simulink model "for_elsa"  (R2020a)
settings: Solver=FixedStepAuto  StartTime=0.0  StopTime=10.0  FixedStep=1e-3  RelTol=1e-3  EnableMultiTasking=on
undefined symbols (not defined in the file): A0, A1, D0, D1, D10, D11, D12, D13, D2, D3, D4, D5, D6, D7, D8, D9, PTA0, PTA1, PTA2, PTB2, PTB23, PTB3, PTB9, PTC16, PTC17, PTC2, PTC3, PTC4, PTD0, PTD1, PTD2, PTD3
libraries: frdmk64flib x22, etargetslib x16, dspstat3 x1
settings Model: ExtModeTrigDuration=5  Creator=Luis  LastModifiedBy=Steven
settings OptimizationCC: EnhancedBackFolding=on  PassReuseOutputArgsAs=Individual arguments  ZeroExternalMemoryAtStartup=off  ZeroInternalMemoryAtStartup=off  MaxStackSize=64  OptimizeBlockOrder=speed  DifferentSizesBufferReuse=on  OptimizationCustomize=off  EfficientTunableParamExpr=on
settings DebuggingCC: ParameterTunabilityLossMsg=error
settings HardwareCC: ProdBitPerPointer=32  ProdBitPerSizeT=32  ProdBitPerPtrDiffT=32  ProdLargestAtomicInteger=Long  ProdLargestAtomicFloat=Double  ProdWordSize=32  ProdHWDeviceType=ARM Compatible->ARM Cortex
settings SFSimCC: MATLABDynamicMemAlloc=off
settings RTWCC: SystemTargetFile=ert.tlc  HardwareBoard=NXP FRDM-K64F  TemplateMakefile=ert_default_tmf  Toolchain=GNU Tools for ARM Embedded Processors
settings CodeAppCC: ForceParamTrailComments=on  IgnoreCustomStorageClasses=off  OperatorAnnotations=on  SimulinkDataObjDesc=on  SFDataObjDesc=on  InsertBlockDesc=on

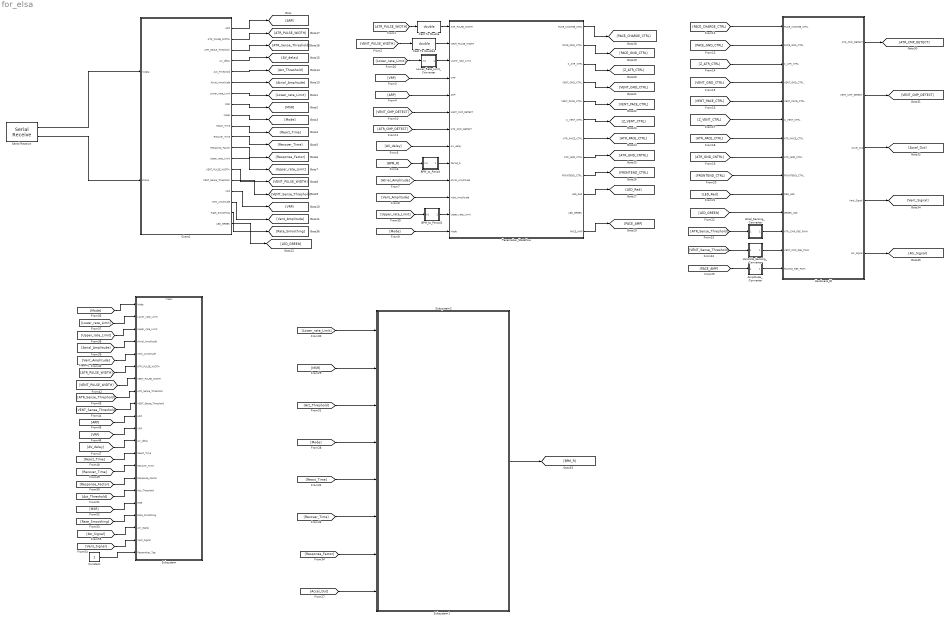
== system for_elsa ==
  Amplitude_Converter : Subsystem
  Atrial_Sensing_Converter : Subsystem
  BPM_to_Period : Subsystem
  BPM_to_Period1 : Subsystem
  Cast To Double : DataTypeConversion  OutDataTypeStr=double
  Cast To Double1 : DataTypeConversion  OutDataTypeStr=double
  Chart1 : Stateflow chart  TreatAsAtomicUnit=on
  Constant : Constant  OutDataTypeStr=uint8
  Hardware_IO : Subsystem
  Lower_Rate_Limit_Converter : Subsystem
  "Pacemaker_Stateflow " : Stateflow chart  TreatAsAtomicUnit=on
      settings: PortSchema="{\"entries\":[{\"content\":{\"sides\":[{\"content\":{\"connectorIds\":[\"In1\",\"In4\",\"In2\",\"In5\",\"In6\",\"In7\",\"In8\",\"In9\",\"In10\",\"In11\",\"In12\",\"In13\",\"In3\"]},\"type\":\"ConnectorPlacement.EquallySpacedRectSide\",\"uuid\":\"f97b12ff-cb00-4386-a373-7143c3a8b48d\"},{\"content\":{\"connectorIds\":[\"Out1\",\"Out2\",\"Out3\",\"Out4\",\"Out5\",\"Out6\",\"Out7\",\"Out8\",\"Out9\",\"Out10\",\"Out11\",\"Out12\"],\"side\":\"RIGHT\"},\"type\":\"ConnectorPlacement.EquallySpacedRectSide\",\"uuid\":\"90163773-f9d1-46de-bd72-9589b8539202\"},{\"content\":{\"connectorIds\":[],\"side\":\"TOP\"},\"type\":\"ConnectorPlacement.EquallySpacedRectSide\",\"uuid\":\"f8a54119-a7c4-4071-8260-df405210e670\"},{\"content\":{\"connectorIds\":[],\"side\":\"BOTTOM\"},\"type\":\"ConnectorPlacement.EquallySpacedRectSide\",\"uuid\":\"70f9d800-d0b8-46e1-812e-9f4712f7acbd\"}]},\"type\":\"ConnectorPlacement.EquallySpacedConnector\",\"uuid\":\"47f7c40c-c42b-42f7-beed-99d299c6cdee\"}],\"packageUris\":[\"http://schema.mathworks.com/mf0/Connector/19700101\"],\"version\":\"1.0\"}"
  Serial Receive : frdmk64flib/Serial Receive  SCIModule=0  Baudrate=uint32(9600)  Parity=None  StopBits=1  HardwareFlowControl=None  ByteOrder=LittleEndian  DataType=uint8  DataLength=37  BlockingMode=off  OutputStatus=on  SampleTime=-1
  Subsystem : Subsystem
  Subsystem1 : Subsystem
  Subsystem2 : Subsystem
  Ventricle_Sensing_Converter : Subsystem
  wires:
  Lower_Rate_Limit_Converter/1(Out1) -> "Pacemaker_Stateflow "/2(Lower_rate_Limit)
  Ventricle_Sensing_Converter/1(Out1) -> Hardware_IO/13(VENT_CMP_REF_PWM)
  Amplitude_Converter/1(Out1) -> Hardware_IO/14(PACING_REF_PWM)
  Atrial_Sensing_Converter/1(Out1) -> Hardware_IO/12(ATR_CMP_REF_PWM)
  Chart1/1(ARP) -> [ARP]
  Chart1/17(Vent_Amplitude) -> [Vent_Amplitude]
  Chart1/16(VRP) -> [VRP]
  Chart1/15(VENT_Sense_Threshold) -> [VENT_Sense_Threshold]
  Chart1/14(VENT_PULSE_WIDTH) -> [VENT_PULSE_WIDTH]
  Chart1/13(Upper_rate_Limit) -> [Upper_rate_Limit]
  Chart1/12(Response_Factor) -> [Response_Factor]
  Chart1/11(Recover_Time) -> [Recover_Time]
  Chart1/10(React_Time) -> [React_Time]
  Chart1/9(Mode) -> [Mode]
  Chart1/8(MSR) -> [MSR]
  Chart1/7(Lower_rate_Limit) -> [Lower_rate_Limit]
  Chart1/5(Act_Threshold) -> [Act_Threshold]
  Chart1/6(Atrial_Amplitude) -> [Atrial_Amplitude]
  Chart1/4(AV_delay) -> [AV_delay]
  Chart1/3(ATR_Sense_Threshold) -> [ATR_Sense_Threshold]
  Chart1/2(ATR_PULSE_WIDTH) -> [ATR_PULSE_WIDTH]
  [Mode] -> "Pacemaker_Stateflow "/3(Mode)
  [Vent_Amplitude] -> "Pacemaker_Stateflow "/12(Vent_Amplitude)
  [Atrial_Amplitude] -> "Pacemaker_Stateflow "/11(Atrial_Amplitude)
  [BPM_R] -> BPM_to_Period/1(In1)
  [AV_delay] -> "Pacemaker_Stateflow "/9(AV_delay)
  [ARP] -> "Pacemaker_Stateflow "/6(ARP)
  [VRP] -> "Pacemaker_Stateflow "/5(VRP)
  [VENT_PULSE_WIDTH] -> Cast To Double1/1
  [ATR_PULSE_WIDTH] -> Cast To Double/1
  [ATR_CMP_DETECT] -> "Pacemaker_Stateflow "/8(ATR_CMP_DETECT)
  [VENT_CMP_DETECT] -> "Pacemaker_Stateflow "/7(VENT_CMP_DETECT)
  "Pacemaker_Stateflow "/1(PACE_CHARGE_CTRL) -> [PACE_CHARGE_CTRL]
  "Pacemaker_Stateflow "/2(PACE_GND_CTRL) -> [PACE_GND_CTRL]
  "Pacemaker_Stateflow "/3(Z_ATR_CTRL) -> [Z_ATR_CTRL]
  "Pacemaker_Stateflow "/4(VENT_GND_CTRL) -> [VENT_GND_CTRL]
  "Pacemaker_Stateflow "/5(VENT_PACE_CTRL) -> [VENT_PACE_CTRL]
  "Pacemaker_Stateflow "/6(Z_VENT_CTRL) -> [Z_VENT_CTRL]
  "Pacemaker_Stateflow "/7(ATR_PACE_CTRL) -> [ATR_PACE_CTRL]
  "Pacemaker_Stateflow "/8(ATR_GND_CTRL) -> [ATR_GND_CNTRL]
  "Pacemaker_Stateflow "/9(FRONTEND_CTRL) -> [FRONTEND_CTRL]
  "Pacemaker_Stateflow "/10(LED_Red) -> [LED_Red]
  "Pacemaker_Stateflow "/12(PACE_AMP) -> [PACE_AMP]
  [PACE_CHARGE_CTRL] -> Hardware_IO/1(PACE_CHARGE_CTRL)
  [PACE_GND_CTRL] -> Hardware_IO/2(PACE_GND_CTRL)
  [Z_ATR_CTRL] -> Hardware_IO/3(Z_ATR_CTRL)
  [VENT_GND_CTRL] -> Hardware_IO/4(VENT_GND_CTRL)
  [VENT_PACE_CTRL] -> Hardware_IO/5(VENT_PACE_CTRL)
  [Z_VENT_CTRL] -> Hardware_IO/6(Z_VENT_CTRL)
  [ATR_PACE_CTRL] -> Hardware_IO/7(ATR_PACE_CTRL)
  [ATR_GND_CNTRL] -> Hardware_IO/8(ATR_GND_CTRL)
  [FRONTEND_CTRL] -> Hardware_IO/9(FRONTEND_CTRL)
  [LED_Red] -> Hardware_IO/10(RED_LED)
  [LED_GREEN] -> Hardware_IO/11(GREEN_LED)
  Hardware_IO/1(ATR_CMP_DETECT) -> [ATR_CMP_DETECT]
  Hardware_IO/2(VENT_CMP_DETECT) -> [VENT_CMP_DETECT]
  [ATR_Sense_Threshold] -> Atrial_Sensing_Converter/1(In1)
  [VENT_Sense_Threshold] -> Ventricle_Sensing_Converter/1(In1)
  [PACE_AMP] -> Amplitude_Converter/1(In1)
  [Lower_rate_Limit] -> Lower_Rate_Limit_Converter/1(In1)
  BPM_to_Period/1(Out1) -> "Pacemaker_Stateflow "/10(Period_R)
  Hardware_IO/3(Accel_Out) -> [Accel_Out]
  [Lower_rate_Limit] -> Subsystem1/1(Lower_Rate)
  [MSR] -> Subsystem1/2(MSR)
  [Act_Threshold] -> Subsystem1/3(Activity_Thresh)
  [React_Time] -> Subsystem1/5(Reaction)
  [Recover_Time] -> Subsystem1/6(Recovery)
  [Response_Factor] -> Subsystem1/7(Response_Factor)
  [Accel_Out] -> Subsystem1/8(Accel_Out)
  Subsystem1/1(BPM_R) -> [BPM_R]
  [Mode] -> Subsystem1/4(Mode)
  Hardware_IO/4(Vent_Signal) -> [Vent_Signal]
  Hardware_IO/5(Atr_Signal) -> [Atr_Signal]
  Serial Receive/2 -> Chart1/2(status)
  Serial Receive/1 -> Chart1/1(rxdata)
  [Upper_rate_Limit] -> BPM_to_Period1/1(In1)
  BPM_to_Period1/1(Out1) -> "Pacemaker_Stateflow "/13(Upper_rate_Limit)
  Chart1/18(Rate_Smoothing) -> [Rate_Smoothing]
  [Mode] -> Subsystem/1(Mode)
  [Lower_rate_Limit] -> Subsystem/2(Lower_rate_Limit)
  [Upper_rate_Limit] -> Subsystem/3(Upper_rate_Limit)
  [Atrial_Amplitude] -> Subsystem/4(Atrial_Amplitude)
  [Vent_Amplitude] -> Subsystem/5(Vent_Amplitude)
  [ATR_PULSE_WIDTH] -> Subsystem/6(ATR_PULSE_WIDTH)
  [VENT_PULSE_WIDTH] -> Subsystem/7(VENT_PULSE_WIDTH)
  [ATR_Sense_Threshold] -> Subsystem/8(ATR_Sense_Threshold)
  [VENT_Sense_Threshold] -> Subsystem/9(VENT_Sense_Threshold)
  [ARP] -> Subsystem/10(ARP)
  [VRP] -> Subsystem/11(VRP)
  [AV_delay] -> Subsystem/12(AV_delay)
  [React_Time] -> Subsystem/13(React_Time)
  [Recover_Time] -> Subsystem/14(Recover_Time)
  [Response_Factor] -> Subsystem/15(Response_Factor)
  [Act_Threshold] -> Subsystem/16(Act_Threshold)
  [MSR] -> Subsystem/17(MSR)
  [Rate_Smoothing] -> Subsystem/18(Rate_Smoothing)
  [Atr_Signal] -> Subsystem/19(Atr_Signal)
  [Vent_Signal] -> Subsystem/20(Vent_Signal)
  Cast To Double/1 -> "Pacemaker_Stateflow "/1(ATR_PULSE_WIDTH)
  Cast To Double1/1 -> "Pacemaker_Stateflow "/4(VENT_PULSE_WIDTH)
  Constant/1 -> Subsystem/21(Pacemaker_Tag)
  Chart1/19(LED_GREEN) -> [LED_GREEN]

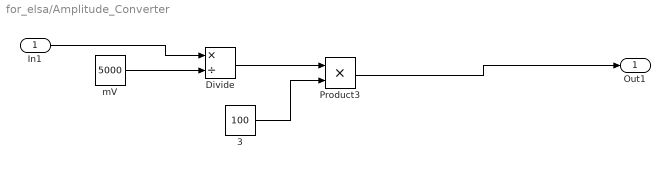
== system for_elsa/Amplitude_Converter ==
  In1 : Inport
  3 : Constant  Value=100  OutDataTypeStr=double
  Divide : Product  Inputs=*/  OutDataTypeStr=double  RndMeth=Nearest
  Product3 : Product  OutDataTypeStr=double
  mV : Constant  Value=5000  OutDataTypeStr=double
  Out1 : Outport
  wires:
  Product3/1 -> Out1/1
  3/1 -> Product3/2
  In1/1 -> Divide/1
  Divide/1 -> Product3/1
  mV/1 -> Divide/2

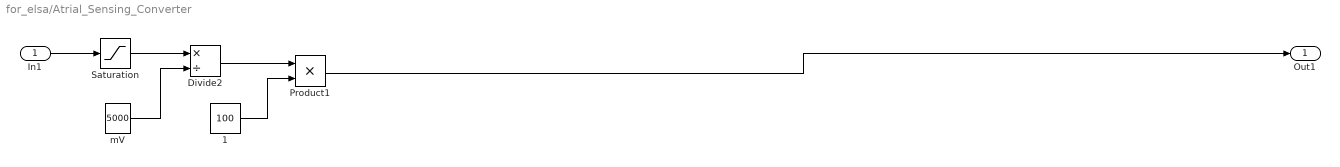
== system for_elsa/Atrial_Sensing_Converter ==
  In1 : Inport
  1 : Constant  Value=100  OutDataTypeStr=uint16
  Divide2 : Product  Inputs=*/  OutDataTypeStr=single
  Product1 : Product  OutDataTypeStr=uint16
  Saturation : Saturate  UpperLimit=4000  LowerLimit=650  LinearizeAsGain=off  OutDataTypeStr=double
  mV : Constant  Value=5000  OutDataTypeStr=double
  Out1 : Outport
  wires:
  Product1/1 -> Out1/1
  1/1 -> Product1/2
  Divide2/1 -> Product1/1
  mV/1 -> Divide2/2
  In1/1 -> Saturation/1
  Saturation/1 -> Divide2/1

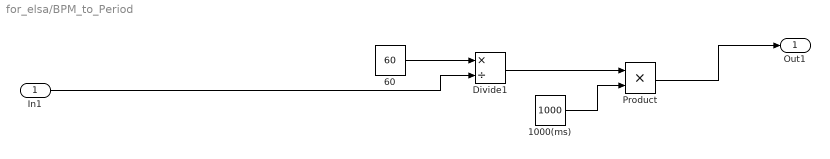
== system for_elsa/BPM_to_Period ==
  In1 : Inport
  1000(ms) : Constant  Value=1000  OutDataTypeStr=uint16
  60 : Constant  Value=60  OutDataTypeStr=uint16
  Divide1 : Product  Inputs=*/
  Product : Product  OutDataTypeStr=uint16
  Out1 : Outport
  wires:
  60/1 -> Divide1/1
  In1/1 -> Divide1/2
  Product/1 -> Out1/1
  Divide1/1 -> Product/1
  1000(ms)/1 -> Product/2

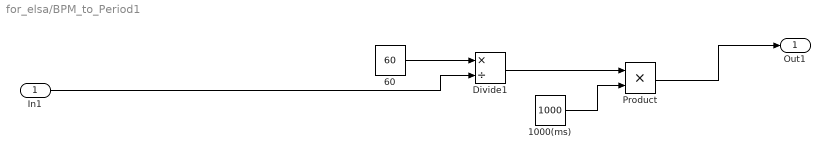
== system for_elsa/BPM_to_Period1 ==
  In1 : Inport
  1000(ms) : Constant  Value=1000  OutDataTypeStr=uint16
  60 : Constant  Value=60  OutDataTypeStr=uint16
  Divide1 : Product  Inputs=*/
  Product : Product  OutDataTypeStr=uint16
  Out1 : Outport
  wires:
  60/1 -> Divide1/1
  In1/1 -> Divide1/2
  Product/1 -> Out1/1
  Divide1/1 -> Product/1
  1000(ms)/1 -> Product/2

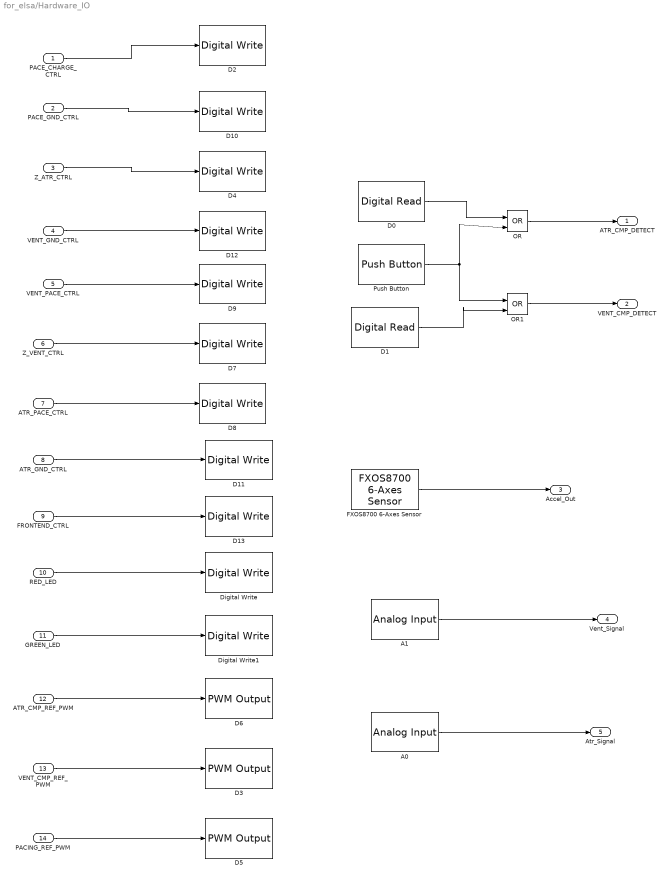
== system for_elsa/Hardware_IO ==
  PACE_CHARGE_CTRL : Inport
  PACE_GND_CTRL : Inport  Port=2
  Z_ATR_CTRL : Inport  Port=3
  VENT_GND_CTRL : Inport  Port=4
  VENT_PACE_CTRL : Inport  Port=5
  Z_VENT_CTRL : Inport  Port=6
  ATR_PACE_CTRL : Inport  Port=7
  ATR_GND_CTRL : Inport  Port=8
  FRONTEND_CTRL : Inport  Port=9
  RED_LED : Inport  Port=10
  GREEN_LED : Inport  Port=11
  ATR_CMP_REF_PWM : Inport  Port=12
  VENT_CMP_REF_PWM : Inport  Port=13
  PACING_REF_PWM : Inport  Port=14
  A0 : frdmk64flib/Analog Input  Whichpin=PTB2 (A0)  SampleTime=-1
  A1 : frdmk64flib/Analog Input  Whichpin=PTB3 (A1)  SampleTime=-1
  D0 : frdmk64flib/Digital Read  Whichpin=PTC16 (D0)  SampleTime=-1
  D1 : frdmk64flib/Digital Read  Whichpin=PTC17 (D1)  SampleTime=-1
  D10 : frdmk64flib/Digital Write  Whichpin=PTD0 (D10)
  D11 : frdmk64flib/Digital Write  Whichpin=PTD2 (D11)
  D12 : frdmk64flib/Digital Write  Whichpin=PTD3 (D12)
  D13 : frdmk64flib/Digital Write  Whichpin=PTD1 (D13)
  D2 : frdmk64flib/Digital Write  Whichpin=PTB9 (D2)
  D3 : frdmk64flib/PWM Output  Whichpin=PTA1 (D3)  InitialFrequency=2000  InitialDutyCycle=0
  D4 : frdmk64flib/Digital Write  Whichpin=PTB23 (D4)
  D5 : frdmk64flib/PWM Output  Whichpin=PTA2 (D5)  InitialFrequency=2000  InitialDutyCycle=0
  D6 : frdmk64flib/PWM Output  Whichpin=PTC2 (D6)  InitialFrequency=2000  InitialDutyCycle=0
  D7 : frdmk64flib/Digital Write  Whichpin=PTC3 (D7)
  D8 : frdmk64flib/Digital Write  Whichpin=PTA0 (D8)
  D9 : frdmk64flib/Digital Write  Whichpin=PTC4 (D9)
  Digital Write : frdmk64flib/Digital Write  Whichpin=RED_LED
  Digital Write1 : frdmk64flib/Digital Write  Whichpin=GREEN_LED
  FXOS8700 6-Axes Sensor : frdmk64flib/FXOS8700 6-Axes Sensor  Activesensor=Accelerometer only  ODR=200Hz  HybridODR=400Hz  Accelfullrange=-4g to +4g  SampleTime=0.01
  OR : Logic  Operator=OR  IconShape=distinctive  AllPortsSameDT=off  OutDataTypeStr=boolean
  OR1 : Logic  Operator=OR  IconShape=distinctive  AllPortsSameDT=off  OutDataTypeStr=boolean
  Push Button : frdmk64flib/Push Button  Whichswitch=SW2  SampleTime1=-1
  ATR_CMP_DETECT : Outport
  VENT_CMP_DETECT : Outport  Port=2
  Accel_Out : Outport  Port=3
  Vent_Signal : Outport  Port=4
  Atr_Signal : Outport  Port=5
  wires:
  PACING_REF_PWM/1 -> D5/1
  RED_LED/1 -> Digital Write/1
  Z_ATR_CTRL/1 -> D4/1
  PACE_CHARGE_CTRL/1 -> D2/1
  VENT_GND_CTRL/1 -> D12/1
  D1/1 -> OR1/2
  ATR_PACE_CTRL/1 -> D8/1
  OR1/1 -> VENT_CMP_DETECT/1
  PACE_GND_CTRL/1 -> D10/1
  ATR_GND_CTRL/1 -> D11/1
  OR/1 -> ATR_CMP_DETECT/1
  D0/1 -> OR/1
  ATR_CMP_REF_PWM/1 -> D6/1
  Push Button/1 -> OR1/1, OR/2
  GREEN_LED/1 -> Digital Write1/1
  FRONTEND_CTRL/1 -> D13/1
  VENT_CMP_REF_PWM/1 -> D3/1
  Z_VENT_CTRL/1 -> D7/1
  VENT_PACE_CTRL/1 -> D9/1
  FXOS8700 6-Axes Sensor/1 -> Accel_Out/1
  A1/1 -> Vent_Signal/1
  A0/1 -> Atr_Signal/1

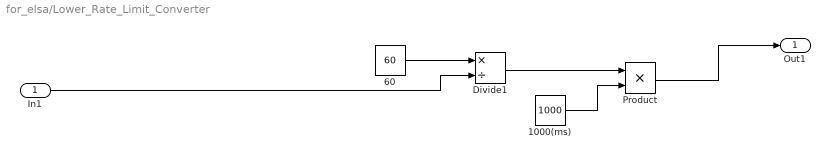
== system for_elsa/Lower_Rate_Limit_Converter ==
  In1 : Inport
  1000(ms) : Constant  Value=1000  OutDataTypeStr=uint16
  60 : Constant  Value=60  OutDataTypeStr=uint16
  Divide1 : Product  Inputs=*/
  Product : Product  OutDataTypeStr=uint16
  Out1 : Outport
  wires:
  60/1 -> Divide1/1
  In1/1 -> Divide1/2
  Product/1 -> Out1/1
  Divide1/1 -> Product/1
  1000(ms)/1 -> Product/2

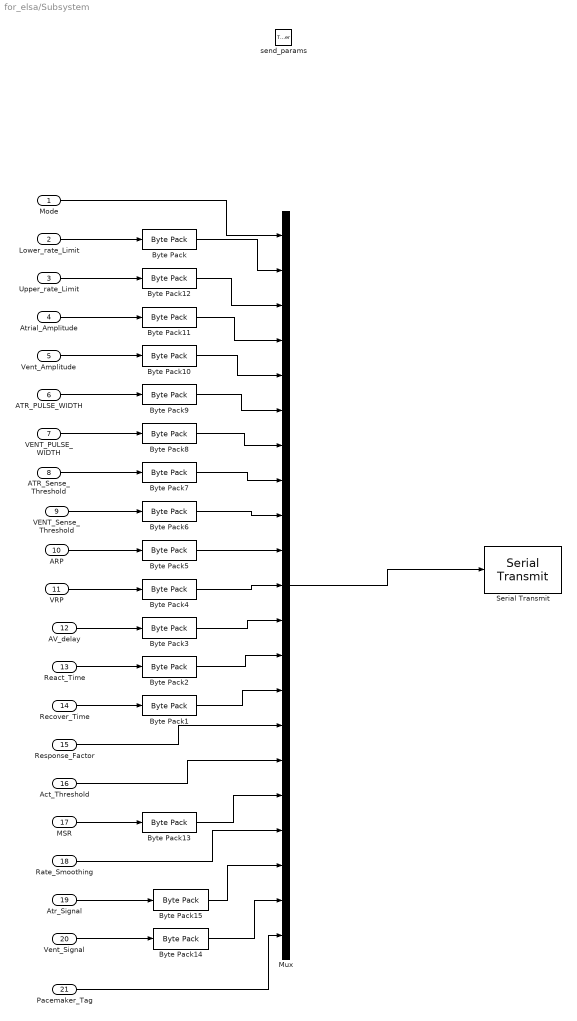
== system for_elsa/Subsystem ==
  Mode : Inport
  Lower_rate_Limit : Inport  Port=2
  Upper_rate_Limit : Inport  Port=3
  Atrial_Amplitude : Inport  Port=4
  Vent_Amplitude : Inport  Port=5
  ATR_PULSE_WIDTH : Inport  Port=6
  VENT_PULSE_WIDTH : Inport  Port=7
  ATR_Sense_Threshold : Inport  Port=8
  VENT_Sense_Threshold : Inport  Port=9
  ARP : Inport  Port=10
  VRP : Inport  Port=11
  AV_delay : Inport  Port=12
  React_Time : Inport  Port=13
  Recover_Time : Inport  Port=14
  Response_Factor : Inport  Port=15
  Act_Threshold : Inport  Port=16
  MSR : Inport  Port=17
  Rate_Smoothing : Inport  Port=18
  Atr_Signal : Inport  Port=19
  Vent_Signal : Inport  Port=20
  Pacemaker_Tag : Inport  Port=21
  send_params : TriggerPort  TriggerType=function-call  IsSimulinkFunction=on  FunctionName=send_params  VariantControl=Variant  PortDimensions=1
  Byte Pack{,1..7,10..13} (12 alike) : etargetslib/Byte Pack  datatypes={'uint16'}  byteAlign=1
  Byte Pack14 : etargetslib/Byte Pack  datatypes={'double'}  byteAlign=1
  Byte Pack15 : etargetslib/Byte Pack  datatypes={'double'}  byteAlign=1
  Byte Pack8 : etargetslib/Byte Pack  datatypes={'single'}  byteAlign=1
  Byte Pack9 : etargetslib/Byte Pack  datatypes={'single'}  byteAlign=1
  Mux : Mux  Inputs=21
  Serial Transmit : frdmk64flib/Serial Transmit  SCIModule=0  Baudrate=uint32(9600)  Parity=None  StopBits=1  HardwareFlowControl=None  ByteOrder=LittleEndian  BlockingMode=on  OutputStatus=off
  wires:
  Mux/1 -> Serial Transmit/1
  Mode/1 -> Mux/1
  Lower_rate_Limit/1 -> Byte Pack/1
  Upper_rate_Limit/1 -> Byte Pack12/1
  Atrial_Amplitude/1 -> Byte Pack11/1
  Vent_Amplitude/1 -> Byte Pack10/1
  ATR_PULSE_WIDTH/1 -> Byte Pack9/1
  VENT_PULSE_WIDTH/1 -> Byte Pack8/1
  ATR_Sense_Threshold/1 -> Byte Pack7/1
  VENT_Sense_Threshold/1 -> Byte Pack6/1
  ARP/1 -> Byte Pack5/1
  VRP/1 -> Byte Pack4/1
  AV_delay/1 -> Byte Pack3/1
  React_Time/1 -> Byte Pack2/1
  Recover_Time/1 -> Byte Pack1/1
  Response_Factor/1 -> Mux/15
  Act_Threshold/1 -> Mux/16
  MSR/1 -> Byte Pack13/1
  Rate_Smoothing/1 -> Mux/18
  Byte Pack/1 -> Mux/2
  Byte Pack12/1 -> Mux/3
  Byte Pack11/1 -> Mux/4
  Byte Pack10/1 -> Mux/5
  Byte Pack9/1 -> Mux/6
  Byte Pack8/1 -> Mux/7
  Byte Pack7/1 -> Mux/8
  Byte Pack6/1 -> Mux/9
  Byte Pack5/1 -> Mux/10
  Byte Pack4/1 -> Mux/11
  Byte Pack3/1 -> Mux/12
  Byte Pack2/1 -> Mux/13
  Byte Pack1/1 -> Mux/14
  Byte Pack13/1 -> Mux/17
  Atr_Signal/1 -> Byte Pack15/1
  Vent_Signal/1 -> Byte Pack14/1
  Byte Pack15/1 -> Mux/19
  Byte Pack14/1 -> Mux/20
  Pacemaker_Tag/1 -> Mux/21

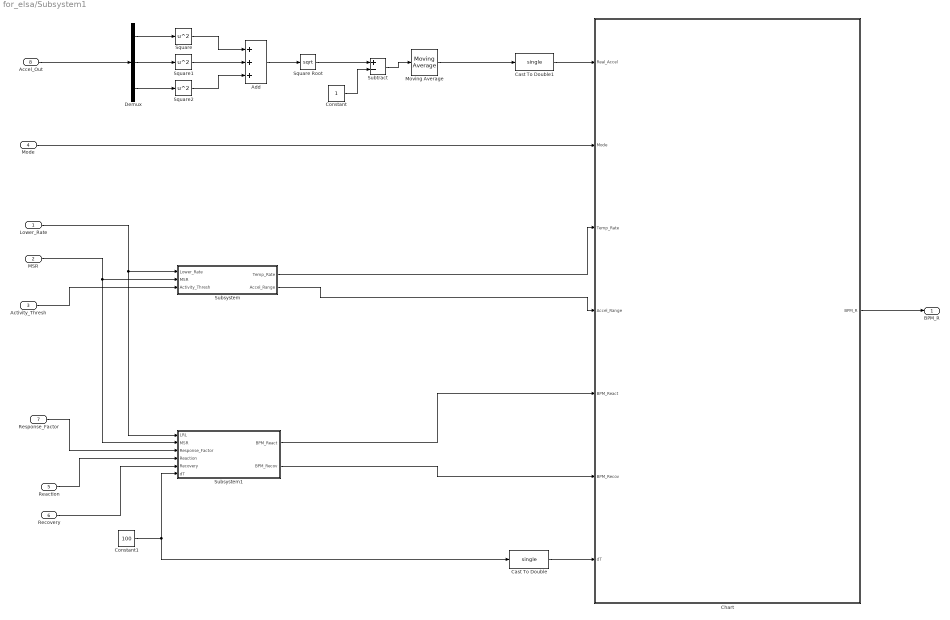
== system for_elsa/Subsystem1 ==
  Lower_Rate : Inport
  MSR : Inport  Port=2
  Activity_Thresh : Inport  Port=3
  Mode : Inport  Port=4
  Reaction : Inport  Port=5
  Recovery : Inport  Port=6
  Response_Factor : Inport  Port=7
  Accel_Out : Inport  Port=8
  Add : Sum  Inputs=+++
  Cast To Double : DataTypeConversion  OutDataTypeStr=single
  Cast To Double1 : DataTypeConversion  OutDataTypeStr=single
  Chart : Stateflow chart  TreatAsAtomicUnit=on
      settings: PortSchema="{\"entries\":[{\"content\":{\"sides\":[{\"content\":{\"connectorIds\":[\"In6\",\"In7\",\"In1\",\"In5\",\"In4\",\"In3\",\"In2\"]},\"type\":\"ConnectorPlacement.EquallySpacedRectSide\",\"uuid\":\"fd37fbd3-e000-4689-ac4c-c5dc5f9ff249\"},{\"content\":{\"connectorIds\":[\"Out1\"],\"side\":\"RIGHT\"},\"type\":\"ConnectorPlacement.EquallySpacedRectSide\",\"uuid\":\"ecd47ea8-5163-45dd-b16f-b562f4f32b7a\"},{\"content\":{\"connectorIds\":[],\"side\":\"TOP\"},\"type\":\"ConnectorPlacement.EquallySpacedRectSide\",\"uuid\":\"5a12f78e-09eb-4424-b8df-032bb9c35282\"}]},\"type\":\"ConnectorPlacement.EquallySpacedConnector\",\"uuid\":\"ee531c1a-9330-4011-aacb-36658e3c3abb\"}],\"packageUris\":[\"http://schema.mathworks.com/mf0/Connector/19700101\"],\"version\":\"1.0\"}"
  Constant : Constant
  Constant1 : Constant  Value=100
  Demux : Demux  Outputs=3
  Moving Average : dspstat3/Moving Average  Method=Sliding window  ForgettingFactorPort=off  SpecifyWindowLength=on  WindowLength=25  ForgettingFactor=0.9  SimulateUsing=Code generation
  Square : Math  Operator=square  SaturateOnIntegerOverflow=on
  Square Root : Sqrt  SaturateOnIntegerOverflow=on
  Square1 : Math  Operator=square  SaturateOnIntegerOverflow=on
  Square2 : Math  Operator=square  SaturateOnIntegerOverflow=on
  Subsystem : Subsystem
  Subsystem1 : Subsystem
  Subtract : Sum  Inputs=+-
  BPM_R : Outport
  wires:
  Demux/3 -> Square2/1
  Subsystem1/1(BPM_React) -> Chart/4(BPM_React)
  Subsystem/1(Temp_Rate) -> Chart/1(Temp_Rate)
  Accel_Out/1 -> Demux/1
  Square/1 -> Add/1
  Demux/2 -> Square1/1
  Mode/1 -> Chart/7(Mode)
  Lower_Rate/1 -> Subsystem/1(Lower_Rate), Subsystem1/1(LRL)
  Response_Factor/1 -> Subsystem1/3(Response_Factor)
  Recovery/1 -> Subsystem1/5(Recovery)
  Add/1 -> Square Root/1
  Subsystem/2(Accel_Range) -> Chart/5(Accel_Range)
  Constant/1 -> Subtract/2
  Subtract/1 -> Moving Average/1
  Square Root/1 -> Subtract/1
  Subsystem1/2(BPM_Recov) -> Chart/3(BPM_Recov)
  Constant1/1 -> Subsystem1/6(dT), Cast To Double/1
  Demux/1 -> Square/1
  Moving Average/1 -> Cast To Double1/1
  Activity_Thresh/1 -> Subsystem/3(Activity_Thresh)
  Square1/1 -> Add/2
  Square2/1 -> Add/3
  Reaction/1 -> Subsystem1/4(Reaction)
  MSR/1 -> Subsystem/2(MSR), Subsystem1/2(MSR)
  Chart/1(BPM_R) -> BPM_R/1
  Cast To Double/1 -> Chart/2(dT)
  Cast To Double1/1 -> Chart/6(Real_Accel)

== system for_elsa/Subsystem2 ==

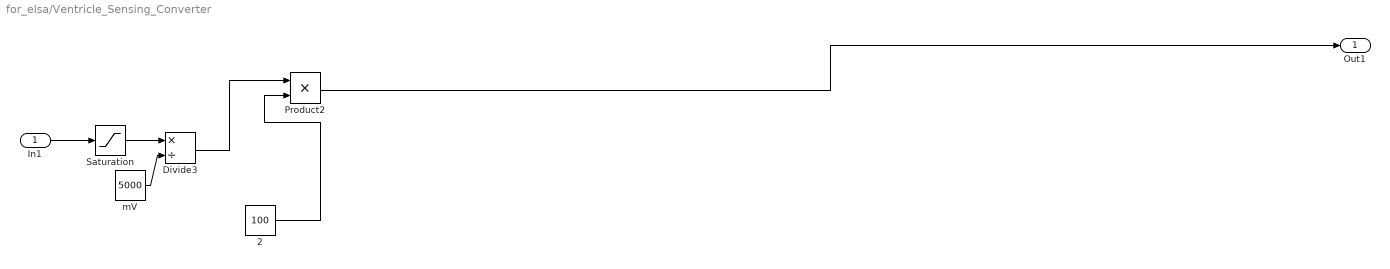
== system for_elsa/Ventricle_Sensing_Converter ==
  In1 : Inport
  2 : Constant  Value=100  OutDataTypeStr=uint16
  Divide3 : Product  Inputs=*/  OutDataTypeStr=single
  Product2 : Product  OutDataTypeStr=uint16
  Saturation : Saturate  UpperLimit=4000  LowerLimit=650  LinearizeAsGain=off  OutDataTypeStr=double
  mV : Constant  Value=5000  OutDataTypeStr=double
  Out1 : Outport
  wires:
  Product2/1 -> Out1/1
  mV/1 -> Divide3/2
  Divide3/1 -> Product2/1
  In1/1 -> Saturation/1
  2/1 -> Product2/2
  Saturation/1 -> Divide3/1

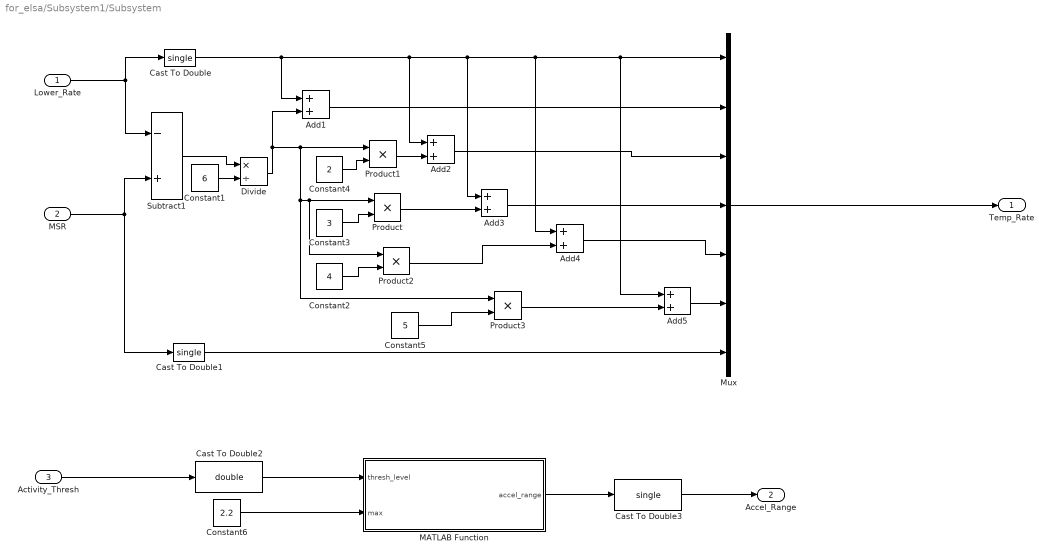
== system for_elsa/Subsystem1/Subsystem ==
  Lower_Rate : Inport
  MSR : Inport  Port=2
  Activity_Thresh : Inport  Port=3
  Add{1,3..5} (4 alike) : Sum  OutDataTypeStr=single
  Add2 : Sum  AccumDataTypeStr=single  OutDataTypeStr=single
  Cast To Double : DataTypeConversion  OutDataTypeStr=single
  Cast To Double1 : DataTypeConversion  OutDataTypeStr=single
  Cast To Double2 : DataTypeConversion  OutDataTypeStr=double
  Cast To Double3 : DataTypeConversion  OutDataTypeStr=single
  Constant1 : Constant  Value=6
  Constant2 : Constant  Value=4
  Constant3 : Constant  Value=3
  Constant4 : Constant  Value=2
  Constant5 : Constant  Value=5
  Constant6 : Constant  Value=2.2  OutDataTypeStr=double
  Divide : Product  Inputs=*/
  MATLAB Function : MATLAB Function  TreatAsAtomicUnit=on
  Mux : Mux  Inputs=7
  Product{,1..3} (4 alike) : Product
  Subtract1 : Sum  Inputs=-+
  Temp_Rate : Outport
  Accel_Range : Outport  Port=2  OutDataTypeStr=single
  wires:
  Constant4/1 -> Product1/2
  Constant1/1 -> Divide/2
  Constant6/1 -> MATLAB Function/2(max)
  Product3/1 -> Add5/2
  MSR/1 -> Cast To Double1/1, Subtract1/2
  Add3/1 -> Mux/4
  Cast To Double/1 -> Add1/1, Mux/1, Add5/1, Add4/1, Add3/1, Add2/1
  Constant3/1 -> Product/2
  Product1/1 -> Add2/2
  Add5/1 -> Mux/6
  Subtract1/1 -> Divide/1
  Activity_Thresh/1 -> Cast To Double2/1
  Divide/1 -> Product3/1, Product2/1, Product/1, Product1/1, Add1/2
  Product2/1 -> Add4/2
  Product/1 -> Add3/2
  Add4/1 -> Mux/5
  Constant2/1 -> Product2/2
  Add2/1 -> Mux/3
  Lower_Rate/1 -> Cast To Double/1, Subtract1/1
  Mux/1 -> Temp_Rate/1
  Cast To Double1/1 -> Mux/7
  Constant5/1 -> Product3/2
  Add1/1 -> Mux/2
  MATLAB Function/1(accel_range) -> Cast To Double3/1
  Cast To Double2/1 -> MATLAB Function/1(thresh_level)
  Cast To Double3/1 -> Accel_Range/1

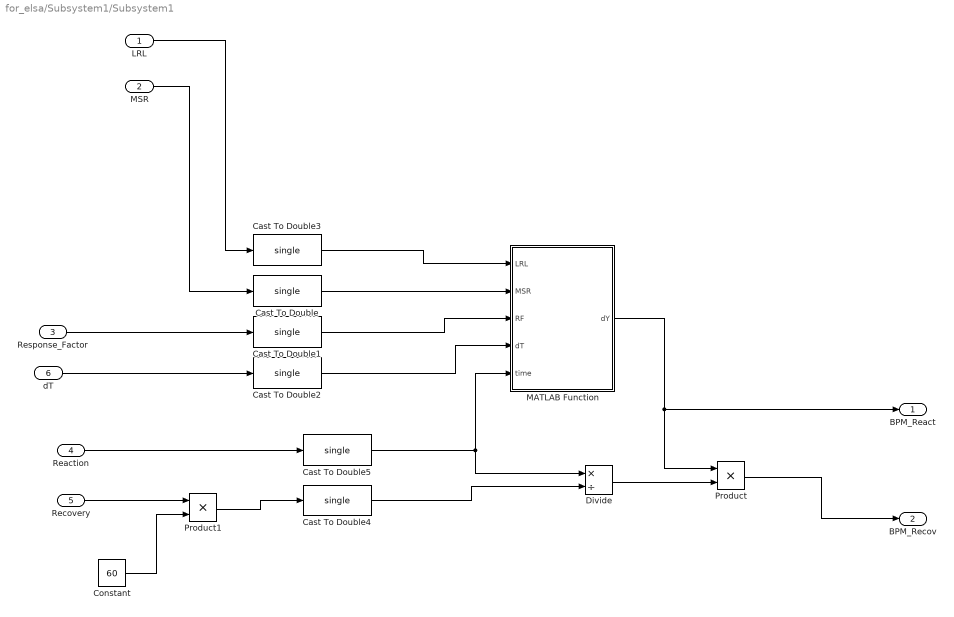
== system for_elsa/Subsystem1/Subsystem1 ==
  LRL : Inport
  MSR : Inport  Port=2
  Response_Factor : Inport  Port=3
  Reaction : Inport  Port=4
  Recovery : Inport  Port=5
  dT : Inport  Port=6
  Cast To Double{,1..5} (6 alike) : DataTypeConversion  OutDataTypeStr=single
  Constant : Constant  Value=60
  Divide : Product  Inputs=*/
  MATLAB Function : MATLAB Function  TreatAsAtomicUnit=on
  Product : Product
  Product1 : Product
  BPM_React : Outport
  BPM_Recov : Outport  Port=2
  wires:
  Product1/1 -> Cast To Double4/1
  Constant/1 -> Product1/2
  Recovery/1 -> Product1/1
  Reaction/1 -> Cast To Double5/1
  Cast To Double5/1 -> MATLAB Function/5(time), Divide/1
  Cast To Double/1 -> MATLAB Function/2(MSR)
  MSR/1 -> Cast To Double/1
  MATLAB Function/1(dY) -> Product/1, BPM_React/1
  Response_Factor/1 -> Cast To Double1/1
  Cast To Double1/1 -> MATLAB Function/3(RF)
  Cast To Double4/1 -> Divide/2
  Cast To Double2/1 -> MATLAB Function/4(dT)
  LRL/1 -> Cast To Double3/1
  Divide/1 -> Product/2
  Cast To Double3/1 -> MATLAB Function/1(LRL)
  dT/1 -> Cast To Double2/1
  Product/1 -> BPM_Recov/1

== stateflow chart for_elsa/Chart1 ==
  settings: executeAtInitialization=1
  state PARAMETER_CHECK
    entry:
    if Lower_rate_Limit < 30 || Lower_rate_Limit > 175||Upper_rate_Limit < 50 || Upper_rate_Limit >175 ...
    || Atrial_Amplitude < 100 || Atrial_Amplitude > 5000 || Vent_Amplitude < 100 || Vent_Amplitude > 5000 ...
    || ATR_PULSE_WIDTH < 1 || ATR_PULSE_WIDTH > 30 || VENT_PULSE_WIDTH < 1 || VENT_PULSE_WIDTH  30 ...
    || ATR_Sense_Threshold < 500 || ATR_Sense_Threshold > 5000 || VENT_Sense_Threshold < 500 || VENT_Sense_Threshold > 5000 ...
    || ARP < 150 || ARP > 500 || VRP < 150 || VRP > 500 ...
    || AV_delay < 70 || AV_delay > 300 || React_Time < 10 || React_Time > 50 ...
    || Recover_Time < 2 ||  Recover_Time > 16 || Response_Factor < 1 || Response_Factor > 16 ...
    || Act_Threshold < 1 || Act_Threshold > 7 || MSR < 50 || MSR > 175 || Rate_Smoothing > 25
    Mode = 0;
    end
  state SET_PARAMS
    entry:
    Mode = rxdata(2);
    Lower_rate_Limit=typecast(rxdata(3:4), 'uint16');
    Upper_rate_Limit=typecast(rxdata(5:6), 'uint16');
    Atrial_Amplitude=typecast(rxdata(7:8), 'uint16');
    Vent_Amplitude=typecast(rxdata(9:10), 'uint16');
    ATR_PULSE_WIDTH=typecast(rxdata(11:14), 'single');
    VENT_PULSE_WIDTH=typecast(rxdata(15:18), 'single');
    ATR_Sense_Threshold=typecast(rxdata(19:20), 'uint16');
    VENT_Sense_Threshold=typecast(rxdata(21:22), 'uint16');
    ARP=typecast(rxdata(23:24), 'uint16');
    VRP=typecast(rxdata(25:26), 'uint16');
    AV_delay=typecast(rxdata(27:28), 'uint16');
    React_Time=typecast(rxdata(29:30), 'uint16');
    Recover_Time=typecast(rxdata(31:32), 'uint16');
    Response_Factor= rxdata(33);
    Act_Threshold=rxdata(34);
    MSR=typecast(rxdata(35:36),'uint16'); %should switch to uint8?
    Rate_Smoothing = rxdata(37);
    send_params();
  state INITIAL
    entry:
    Mode = 0;
    Lower_rate_Limit=70;
    Atrial_Amplitude=5000;
    Vent_Amplitude=5000;
    ATR_PULSE_WIDTH=1;
    VENT_PULSE_WIDTH=1;
    ATR_Sense_Threshold=2750;
    VENT_Sense_Threshold=2750;
    ARP=250;
    VRP=320;
    AV_delay=100;
    React_Time=40;
    Recover_Time=5;
    Response_Factor=16;
    Act_Threshold=7;
    MSR=120;
    Rate_Smoothing = 0;
  state STANBY
    %Waiting for COM
  state EGRAM
    entry:
    LED_GREEN = true;
    send_params();
  SET_PARAMS -> PARAMETER_CHECK
  PARAMETER_CHECK -> STANBY
  (junction 11) -> SET_PARAMS [order 1] : [rxdata(1) == 0x00]
  (default) -> INITIAL
  STANBY -> (junction 11) : [status ==0 ]
  (junction 11) -> EGRAM [order 2] : [rxdata(1) > 0x01]
  INITIAL -> STANBY
  EGRAM -> STANBY
  data: rxdata input uint8; ARP output uint16; ATR_PULSE_WIDTH output single; ATR_Sense_Threshold output uint16; status input uint8; AV_delay output uint16; Act_Threshold output uint8; Atrial_Amplitude output uint16; Lower_rate_Limit output uint16; MSR output uint16; Mode output uint8; React_Time output uint16; Recover_Time output uint16; Response_Factor output uint8; Upper_rate_Limit output uint16; VENT_PULSE_WIDTH output single; VENT_Sense_Threshold output uint16; VRP output uint16; Vent_Amplitude output uint16; Rate_Smoothing output uint8; LED_GREEN output boolean

== stateflow chart for_elsa/Pacemaker_Stateflow  ==
  state AOO
    state AOO_CHARGING
      entry:
      %Charge C22
      ATR_PACE_CTRL=false;
      VENT_PACE_CTRL=false;
      PACE_CHARGE_CTRL=true;
      %Discharge C21
      PACE_GND_CTRL=true;
      Z_VENT_CTRL=false;
      Z_ATR_CTRL=false;
      ATR_GND_CTRL=true;
      PACE_AMP = Atrial_Amplitude;
      VENT_GND_CTRL=false;
      LED_Red = false;
    state AOO_DISCHARGING
      entry:
      %Discharge C22 into ATR
      %Charge C21
      PACE_CHARGE_CTRL=false;
      PACE_GND_CTRL=true;
      ATR_PACE_CTRL=true;
      ATR_GND_CTRL=false;
      Z_VENT_CTRL=false;
      Z_ATR_CTRL=false;
      VENT_GND_CTRL=false;
      VENT_PACE_CTRL=false;
      LED_Red = true;
    AOO_DISCHARGING -> AOO_CHARGING : after(ATR_PULSE_WIDTH,msec)
    AOO_CHARGING -> AOO_DISCHARGING [order 2] : after(Lower_rate_Limit - ATR_PULSE_WIDTH,msec)
  state DOOR [group]
    state DOOR_CHARGING_V
      entry:
      %Charge C22
      VENT_PACE_CTRL=false;
      ATR_PACE_CTRL=false;
      PACE_CHARGE_CTRL=true;
      %Discharge C21 to V
      PACE_GND_CTRL=true;
      Z_VENT_CTRL=false;
      Z_ATR_CTRL=false;
      ATR_PACE_CTRL=false;
      ATR_GND_CTRL=false;
      VENT_GND_CTRL=true;
      LED_GREEN = false;
      %Set PACING_REF_PWM
      PACE_AMP=Atrial_Amplitude;
    state DOOR_PACE_A
      entry:
      %Discharge C22 into ATR
      %Charge C21
      PACE_CHARGE_CTRL=false;
      PACE_GND_CTRL=true;
      ATR_PACE_CTRL=true;
      ATR_GND_CTRL=false;
      Z_VENT_CTRL=false;
      Z_ATR_CTRL=false;
      VENT_GND_CTRL=false;
      VENT_PACE_CTRL=false;
      LED_Red = true;
    state DOOR_CHARGING_A
      entry:
      %Charge C22
      ATR_PACE_CTRL=false;
      VENT_PACE_CTRL=false;
      PACE_CHARGE_CTRL=true;
      %Discharge C21
      PACE_GND_CTRL=true;
      Z_VENT_CTRL=false;
      Z_ATR_CTRL=false;
      ATR_GND_CTRL=true;
      VENT_GND_CTRL=false;
      LED_Red = false;
      %Set PACING_REF_PWM
      PACE_AMP=Vent_Amplitude
    state DOOR_PACE_V
      entry:
      %Discharge C22 into VENT
      %Charge C21
      PACE_CHARGE_CTRL=false;
      PACE_GND_CTRL=true;
      ATR_PACE_CTRL=false;
      ATR_GND_CTRL=false;
      Z_ATR_CTRL=false
      Z_VENT_CTRL=false;
      VENT_GND_CTRL=false;
      VENT_PACE_CTRL=true;
      LED_GREEN = true;
    DOOR_CHARGING_V -> DOOR_PACE_A [order 2] : after(Period_R - (AV_delay+VENT_PULSE_WIDTH),msec)
    DOOR_PACE_V -> DOOR_CHARGING_V : after(VENT_PULSE_WIDTH, msec)
    DOOR_PACE_A -> DOOR_CHARGING_A : after(ATR_PULSE_WIDTH,msec)
    DOOR_CHARGING_A -> DOOR_PACE_V : after(AV_delay - ATR_PULSE_WIDTH,msec)
  state VOO [group]
    state VOO_DISCHARGE
      entry:
      %Discharge C22 into VENT
      %Charge C21
      PACE_CHARGE_CTRL=false;
      PACE_GND_CTRL=true;
      ATR_PACE_CTRL=false;
      ATR_GND_CTRL=false;
      Z_ATR_CTRL=false
      Z_VENT_CTRL=false;
      VENT_GND_CTRL=false;
      VENT_PACE_CTRL=true;
      LED_GREEN = true;
    state VOO_CHARGING
      entry:
      %Charge C22
      VENT_PACE_CTRL=false;
      ATR_PACE_CTRL=false;
      PACE_CHARGE_CTRL=true;
      %Discharge C21
      PACE_GND_CTRL=true;
      Z_VENT_CTRL=false;
      Z_ATR_CTRL=false;
      ATR_PACE_CTRL=false;
      ATR_GND_CTRL=false;
      PACE_AMP = Vent_Amplitude;
      VENT_GND_CTRL=true;
      LED_GREEN = false;
    VOO_DISCHARGE -> VOO_CHARGING : after(VENT_PULSE_WIDTH, msec)
    VOO_CHARGING -> VOO_DISCHARGE [order 2] : after(Lower_rate_Limit - VENT_PULSE_WIDTH, msec)
  state VVIR [group]
    state VVIR_CHARGING
      entry:
      FRONTEND_CTRL = true;
      PACE_GND_CTRL = true;
      VENT_PACE_CTRL=false;
      ATR_PACE_CTRL=false;
      PACE_CHARGE_CTRL=true;
      Z_VENT_CTRL=false;
      Z_ATR_CTRL=false;
      ATR_GND_CTRL=false;
      PACE_AMP = Vent_Amplitude;
      VENT_GND_CTRL=true;
      LED_GREEN = false;
    state VIIR_VENTRICAL_PACE
      entry:
      FRONTEND_CTRL = false;
      PACE_GND_CTRL = true;
      VENT_PACE_CTRL=true;
      ATR_PACE_CTRL=false;
      PACE_CHARGE_CTRL=false;
      Z_VENT_CTRL=false;
      Z_ATR_CTRL=false;
      ATR_GND_CTRL=false;
      VENT_GND_CTRL=false;
      LED_GREEN = true;
    state VVIR_VRP
      entry:
      PACE_GND_CTRL = true;
      VENT_PACE_CTRL=false;
      ATR_PACE_CTRL=false;
      PACE_CHARGE_CTRL=true;
      Z_VENT_CTRL=false;
      Z_ATR_CTRL=false;
      ATR_GND_CTRL=false;
      VENT_GND_CTRL=true;
      LED_GREEN = false;
    VVIR_CHARGING -> VIIR_VENTRICAL_PACE [order 2] : after(Period_R - (VENT_PULSE_WIDTH + VRP), msec)
    VVIR_CHARGING -> VVIR_VRP [order 3] : [VENT_CMP_DETECT == true]
    VVIR_VRP -> VVIR_CHARGING : after(VRP, msec)
    VIIR_VENTRICAL_PACE -> VVIR_VRP : after(VENT_PULSE_WIDTH, msec)
  state VVI [group]
    state VII_CHARGING
      entry:
      FRONTEND_CTRL = true;
      PACE_GND_CTRL = true;
      VENT_PACE_CTRL=false;
      ATR_PACE_CTRL=false;
      PACE_CHARGE_CTRL=true;
      Z_VENT_CTRL=false;
      Z_ATR_CTRL=false;
      ATR_GND_CTRL=false;
      PACE_AMP = Vent_Amplitude;
      VENT_GND_CTRL=true;
      LED_GREEN = false;
    state VII_VENTRICAL_PACE
      entry:
      FRONTEND_CTRL = false;
      PACE_GND_CTRL = true;
      VENT_PACE_CTRL=true;
      ATR_PACE_CTRL=false;
      PACE_CHARGE_CTRL=false;
      Z_VENT_CTRL=false;
      Z_ATR_CTRL=false;
      ATR_GND_CTRL=false;
      VENT_GND_CTRL=false;
      LED_GREEN = true;
    state VII_VRP
      entry:
      PACE_GND_CTRL = true;
      VENT_PACE_CTRL=false;
      ATR_PACE_CTRL=false;
      PACE_CHARGE_CTRL=true;
      Z_VENT_CTRL=false;
      Z_ATR_CTRL=false;
      ATR_GND_CTRL=false;
      VENT_GND_CTRL=true;
      LED_GREEN = false;
    VII_CHARGING -> VII_VENTRICAL_PACE [order 3] : after((Lower_rate_Limit) - (VENT_PULSE_WIDTH + VRP), msec)
    VII_CHARGING -> VII_VRP [order 2] : [VENT_CMP_DETECT == true]
    VII_VRP -> VII_CHARGING : after(VRP, msec)
    VII_VENTRICAL_PACE -> VII_VRP : after(VENT_PULSE_WIDTH, msec)
  state Default
    entry:
    %Charge C22
    ATR_PACE_CTRL=false;
    VENT_PACE_CTRL=false;
    PACE_CHARGE_CTRL=false;
    %Discharge C21
    PACE_GND_CTRL=false;
    Z_VENT_CTRL=false;
    Z_ATR_CTRL=false;
    ATR_GND_CTRL=false;
    VENT_GND_CTRL=false;
    FRONTEND_CTRL=true;
    LED_Red=false;
    LED_GREEN=false;
  state AAIR [group]
    state AAIR_CHARGING
      entry:
      FRONTEND_CTRL = true;
      PACE_GND_CTRL = true;
      VENT_PACE_CTRL=false;
      ATR_PACE_CTRL=false;
      PACE_CHARGE_CTRL=true;
      Z_VENT_CTRL=false;
      Z_ATR_CTRL=false;
      ATR_GND_CTRL=true;
      PACE_AMP = Atrial_Amplitude;
      VENT_GND_CTRL=false;
      LED_Red = false;
    state AAIR_ATRIAL_PACE
      entry:
      FRONTEND_CTRL = false;
      PACE_GND_CTRL = true;
      VENT_PACE_CTRL=false;
      ATR_PACE_CTRL=true;
      PACE_CHARGE_CTRL=false;
      Z_VENT_CTRL=false;
      Z_ATR_CTRL=false;
      ATR_GND_CTRL=false;
      VENT_GND_CTRL=false;
      LED_Red = true;
    state AAIR_ARP
      entry:
      PACE_GND_CTRL = true;
      VENT_PACE_CTRL=false;
      ATR_PACE_CTRL=false;
      PACE_CHARGE_CTRL=true;
      Z_VENT_CTRL=false;
      Z_ATR_CTRL=false;
      ATR_GND_CTRL=true;
      VENT_GND_CTRL=false;
      LED_Red = false;
    AAIR_CHARGING -> AAIR_ATRIAL_PACE [order 2] : after((Period_R) - (ATR_PULSE_WIDTH + ARP), msec)
    AAIR_CHARGING -> AAIR_ARP [order 3] : [ATR_CMP_DETECT == true]
    AAIR_ARP -> AAIR_CHARGING : after(ARP, msec)
    AAIR_ATRIAL_PACE -> AAIR_ARP : after(ATR_PULSE_WIDTH, msec)
  state AAI [group]
    state AII_CHARGING
      entry:
      FRONTEND_CTRL = true;
      PACE_GND_CTRL = true;
      VENT_PACE_CTRL=false;
      ATR_PACE_CTRL=false;
      PACE_CHARGE_CTRL=true;
      Z_VENT_CTRL=false;
      Z_ATR_CTRL=false;
      ATR_GND_CTRL=true;
      PACE_AMP = Atrial_Amplitude;
      VENT_GND_CTRL=false;
      LED_Red = false;
    state AII_ATRIAL_PACE
      entry:
      FRONTEND_CTRL = false;
      PACE_GND_CTRL = true;
      VENT_PACE_CTRL=false;
      ATR_PACE_CTRL=true;
      PACE_CHARGE_CTRL=false;
      Z_VENT_CTRL=false;
      Z_ATR_CTRL=false;
      ATR_GND_CTRL=false;
      VENT_GND_CTRL=false;
      LED_Red = true;
    state AII_ARP
      entry:
      PACE_GND_CTRL = true;
      VENT_PACE_CTRL=false;
      ATR_PACE_CTRL=false;
      PACE_CHARGE_CTRL=true;
      Z_VENT_CTRL=false;
      Z_ATR_CTRL=false;
      ATR_GND_CTRL=true;
      VENT_GND_CTRL=false;
      LED_Red = false;
    AII_CHARGING -> AII_ATRIAL_PACE [order 2] : after((Lower_rate_Limit) - (ATR_PULSE_WIDTH + ARP), msec)
    AII_CHARGING -> AII_ARP [order 3] : [ATR_CMP_DETECT == true]
    AII_ARP -> AII_CHARGING : after(ARP, msec)
    AII_ATRIAL_PACE -> AII_ARP : after(ATR_PULSE_WIDTH, msec)
  state VOOR [group]
    state VOOR_CHARGING
      entry:
      %Charge C22
      VENT_PACE_CTRL=false;
      ATR_PACE_CTRL=false;
      PACE_CHARGE_CTRL=true;
      %Discharge C21
      PACE_GND_CTRL=true;
      Z_VENT_CTRL=false;
      Z_ATR_CTRL=false;
      ATR_PACE_CTRL=false;
      ATR_GND_CTRL=false;
      PACE_AMP = Vent_Amplitude;
      VENT_GND_CTRL=true;
      LED_GREEN = false;
    state VOOR_DISCHARGE
      entry:
      %Discharge C22 into VENT
      %Charge C21
      PACE_CHARGE_CTRL=false;
      PACE_GND_CTRL=true;
      ATR_PACE_CTRL=false;
      ATR_GND_CTRL=false;
      Z_ATR_CTRL=false
      Z_VENT_CTRL=false;
      VENT_GND_CTRL=false;
      VENT_PACE_CTRL=true;
      LED_GREEN = true;
    VOOR_DISCHARGE -> VOOR_CHARGING : after(VENT_PULSE_WIDTH, msec)
    VOOR_CHARGING -> VOOR_DISCHARGE [order 2] : after(Period_R - VENT_PULSE_WIDTH, msec)
  state DOO [group]
    state DOO_CHARGING_V
      entry:
      %Charge C22
      VENT_PACE_CTRL=false;
      ATR_PACE_CTRL=false;
      PACE_CHARGE_CTRL=true;
      %Discharge C21 to V
      PACE_GND_CTRL=true;
      Z_VENT_CTRL=false;
      Z_ATR_CTRL=false;
      ATR_PACE_CTRL=false;
      ATR_GND_CTRL=false;
      VENT_GND_CTRL=true;
      LED_GREEN = false;
      %Set PACING_REF_PWM
      PACE_AMP=Atrial_Amplitude;
    state DOO_PACE_A
      entry:
      %Discharge C22 into ATR
      %Charge C21
      PACE_CHARGE_CTRL=false;
      PACE_GND_CTRL=true;
      ATR_PACE_CTRL=true;
      ATR_GND_CTRL=false;
      Z_VENT_CTRL=false;
      Z_ATR_CTRL=false;
      VENT_GND_CTRL=false;
      VENT_PACE_CTRL=false;
      LED_Red = true;
    state DOO_CHARGING_A
      entry:
      %Charge C22
      ATR_PACE_CTRL=false;
      VENT_PACE_CTRL=false;
      PACE_CHARGE_CTRL=true;
      %Discharge C21
      PACE_GND_CTRL=true;
      Z_VENT_CTRL=false;
      Z_ATR_CTRL=false;
      ATR_GND_CTRL=true;
      VENT_GND_CTRL=false;
      LED_Red = false;
      %Set PACING_REF_PWM
      PACE_AMP=Vent_Amplitude
    state DOO_PACE_V
      entry:
      %Discharge C22 into VENT
      %Charge C21
      PACE_CHARGE_CTRL=false;
      PACE_GND_CTRL=true;
      ATR_PACE_CTRL=false;
      ATR_GND_CTRL=false;
      Z_ATR_CTRL=false
      Z_VENT_CTRL=false;
      VENT_GND_CTRL=false;
      VENT_PACE_CTRL=true;
      LED_GREEN = true;
    DOO_CHARGING_V -> DOO_PACE_A [order 2] : after(Lower_rate_Limit-(AV_delay+VENT_PULSE_WIDTH),msec)
    DOO_PACE_A -> DOO_CHARGING_A : after(ATR_PULSE_WIDTH,msec)
    DOO_PACE_V -> DOO_CHARGING_V : after(VENT_PULSE_WIDTH, msec)
    DOO_CHARGING_A -> DOO_PACE_V : after(AV_delay - ATR_PULSE_WIDTH,msec)
  state AOOR
    state AOOR_CHARGING
      entry:
      %Charge C22
      ATR_PACE_CTRL=false;
      VENT_PACE_CTRL=false;
      PACE_CHARGE_CTRL=true;
      %Discharge C21
      PACE_GND_CTRL=true;
      Z_VENT_CTRL=false;
      Z_ATR_CTRL=false;
      ATR_GND_CTRL=true;
      PACE_AMP = Atrial_Amplitude;
      VENT_GND_CTRL=false;
      LED_Red = false;
    state AOOR_DISCHARGING
      entry:
      %Discharge C22 into ATR
      %Charge C21
      PACE_CHARGE_CTRL=false;
      PACE_GND_CTRL=true;
      ATR_PACE_CTRL=true;
      ATR_GND_CTRL=false;
      Z_VENT_CTRL=false;
      Z_ATR_CTRL=false;
      VENT_GND_CTRL=false;
      VENT_PACE_CTRL=false;
      LED_Red = true;
    (default) -> AOOR_CHARGING
    AOOR_CHARGING -> AOOR_DISCHARGING [order 2] : after(Period_R - ATR_PULSE_WIDTH,msec)
    AOOR_DISCHARGING -> AOOR_CHARGING : after(ATR_PULSE_WIDTH,msec)
  Default -> DOOR_CHARGING_V [order 8] : [Mode == 10]
  DOOR_CHARGING_V -> Default [order 1] : [Mode~=10]
  Default -> AOO_CHARGING [order 1] : [Mode == 1]
  AOO_CHARGING -> Default [order 1] : [Mode~=1]
  Default -> VOO_CHARGING [order 2] : [Mode == 2]
  VOO_CHARGING -> Default [order 1] : [Mode~=2]
  Default -> VVIR_CHARGING [order 9] : [Mode ==9]
  VVIR_CHARGING -> Default [order 1] : [Mode ~= 9]
  Default -> VII_CHARGING [order 3] : [Mode == 3]
  VII_CHARGING -> Default [order 1] : [Mode ~= 3]
  (default) -> Default
  Default -> Default [order 11] : [Mode == 0 || Lower_rate_Limit>Upper_rate_Limit]
  Default -> AAIR_CHARGING [order 10] : [Mode == 8]
  AAIR_CHARGING -> Default [order 1] : [Mode ~= 8]
  Default -> AII_CHARGING [order 4] : [Mode == 4]
  AII_CHARGING -> Default [order 1] : [Mode ~= 4]
  Default -> VOOR_CHARGING [order 7] : [Mode == 7]
  VOOR_CHARGING -> Default [order 1] : [Mode ~= 7]
  Default -> AOOR_CHARGING [order 6] : [Mode == 6]
  AOOR_CHARGING -> Default [order 1] : [Mode ~=6]
  DOO_CHARGING_V -> Default [order 1] : [Mode ~= 5]
  Default -> DOO_CHARGING_V [order 5] : [Mode == 5]
  data: PACE_CHARGE_CTRL output boolean; PACE_GND_CTRL output boolean; Z_ATR_CTRL output boolean; VENT_GND_CTRL output boolean; VENT_PACE_CTRL output boolean; Z_VENT_CTRL output boolean; ATR_PULSE_WIDTH input double; Lower_rate_Limit input uint16; Mode input uint8; ATR_PACE_CTRL output boolean; ATR_GND_CTRL output boolean; VENT_PULSE_WIDTH input double; VRP input uint16; ARP input uint16; FRONTEND_CTRL output boolean; VENT_CMP_DETECT input boolean; ATR_CMP_DETECT input boolean; LED_Red output boolean; LED_GREEN output boolean; AV_delay input uint16; Period_R input uint16; Atrial_Amplitude input uint16; Vent_Amplitude input uint16; PACE_AMP output uint16; Upper_rate_Limit input uint16

== stateflow chart for_elsa/Subsystem1/Chart ==
  state A
    entry:
    BPM_R = BPM_R + BPM_React;
  state A1
    entry:
    BPM_R = BPM_R + BPM_React;
  state A5
    entry:
    BPM_R = BPM_R + BPM_React;
  state HIGH
    entry:
    if abs (Temp_Rate(6) - BPM_R)  < 1.0
    BPM_R = Temp_Rate(6);
    end
  state S
    entry:
    BPM_R = BPM_R - BPM_Recov
  state MED_H
    entry:
    if abs (Temp_Rate(5) - BPM_R)  < 1.0
    BPM_R = Temp_Rate(5);
    end
  state S1
    entry:
    BPM_R = BPM_R - BPM_Recov;
  state V_HIGH
    entry:
    if abs (Temp_Rate(7) - BPM_R)  < 1.0
    BPM_R = Temp_Rate(7);
    end
  state A2
    entry:
    BPM_R = BPM_R + BPM_React;
  state MED
    entry:
    if abs (Temp_Rate(4) - BPM_R)  < 1.0
    BPM_R = Temp_Rate(4);
    end
  state S2
    entry:
    BPM_R = BPM_R - BPM_Recov;
  state Init
    entry:
    BPM_R = Temp_Rate(1);
  state M_LOW
    entry:
    if abs (Temp_Rate(3) - BPM_R)  < 1.0
    BPM_R = Temp_Rate(3);
    end
  state A3
    entry:
    BPM_R = BPM_R + BPM_React;
  state V_LOW
    entry:
    if abs (Temp_Rate(1) - BPM_R)  < 1.0
    BPM_R = Temp_Rate(1);
    end
  state S3
    entry:
    BPM_R = BPM_R - BPM_Recov;
  state LOW
    entry:
    if abs (Temp_Rate(2) - BPM_R)  < 1.0
    BPM_R = Temp_Rate(2);
    end
  state S5
    entry:
    BPM_R = BPM_R - BPM_Recov;
  state A4
    entry:
    BPM_R = BPM_R + BPM_React;
  state S4
    entry:
    BPM_R = BPM_R - BPM_Recov;
  A -> HIGH
  HIGH -> A [order 3] : [after(dT,msec) && Temp_Rate(6)>BPM_R]
  A1 -> MED_H
  MED_H -> A1 [order 3] : [after(dT,msec) && Temp_Rate(5)>BPM_R]
  V_HIGH -> A5 [order 2] : [after(dT,msec) && Temp_Rate(7)>BPM_R]
  MED_H -> S1 [order 2] : [after(dT,msec) && Temp_Rate(5)<BPM_R]
  HIGH -> S [order 2] : [after(dT,msec) && Temp_Rate(6)<BPM_R]
  S1 -> MED_H
  S -> HIGH
  HIGH -> (junction 30) [order 1] : [Real_Accel<Accel_Range(5) || Real_Accel>Accel_Range(6)]
  (junction 30) -> HIGH [order 2] : [Real_Accel>Accel_Range(5)]
  MED_H -> (junction 30) [order 1] : [Real_Accel<Accel_Range(4) || Real_Accel>Accel_Range(5)]
  (junction 30) -> MED_H [order 3] : [Real_Accel>Accel_Range(4)]
  (junction 30) -> V_HIGH [order 1] : [Real_Accel>Accel_Range(6)]
  V_HIGH -> (junction 30) [order 1] : [Real_Accel<Accel_Range(6)]
  A2 -> MED
  MED -> A2 [order 3] : [after(dT,msec) && Temp_Rate(4)>BPM_R]
  MED -> S2 [order 2] : [after(dT,msec) && Temp_Rate(4)<BPM_R]
  MED -> (junction 30) [order 1] : [Real_Accel<Accel_Range(3) || Real_Accel>Accel_Range(4)]
  S2 -> MED
  (junction 30) -> MED [order 4] : [Real_Accel>Accel_Range(3)]
  (default) -> Init
  Init -> (junction 30) : [Mode >= 6]
  (junction 30) -> Init [order 8] : [Mode <6]
  V_LOW -> (junction 30) [order 1] : [Real_Accel>Accel_Range(1)]
  M_LOW -> (junction 30) [order 1] : [Real_Accel<Accel_Range(2) || Real_Accel>Accel_Range(3)]
  (junction 30) -> M_LOW [order 5] : [Real_Accel>Accel_Range(2)]
  (junction 30) -> V_LOW [order 7] : [Real_Accel>0]
  LOW -> (junction 30) [order 1] : [Real_Accel<Accel_Range(1) || Real_Accel>Accel_Range(2)]
  (junction 30) -> LOW [order 6] : [Real_Accel>Accel_Range(1)]
  A3 -> M_LOW
  M_LOW -> A3 [order 3] : [after(dT,msec) && Temp_Rate(3)>BPM_R]
  M_LOW -> S3 [order 2] : [after(dT,msec) && Temp_Rate(3)<BPM_R]
  S3 -> M_LOW
  V_LOW -> S5 [order 2] : [after(dT,msec) && Temp_Rate(1)<BPM_R]
  S5 -> V_LOW
  A4 -> LOW
  LOW -> A4 [order 3] : [after(dT,msec) && Temp_Rate(2)>BPM_R]
  LOW -> S4 [order 2] : [after(dT,msec) && Temp_Rate(2)<BPM_R]
  S4 -> LOW
  data: Temp_Rate input single; dT input single; BPM_Recov input single; BPM_React input single; Accel_Range input single; Real_Accel input single; BPM_R output single; Mode input uint8

== matlab function for_elsa/Subsystem1/Subsystem/MATLAB Function ==
  data: thresh_level input; accel_range output; max input
function accel_range = fcn(thresh_level, max)
if thresh_level == 2
    AT =0.4;
elseif thresh_level == 3
    AT =0.6 ;
elseif thresh_level == 4
    AT = 0.8;
elseif thresh_level == 5
    AT =1.0 ;
elseif thresh_level == 6
    AT = 1.2;
elseif thresh_level == 7
    AT = 1.4;
else 
    AT = 0.2;
end
AT1 = (max - AT)*(1/6) + AT;
AT2 = (max - AT)*(2/6) + AT;
AT3 = (max - AT)*(3/6) + AT;
AT4 = (max - AT)*(4/6) + AT;
AT5 = (max - AT)*(5/6) + AT;

accel_range = [AT, AT1, AT2, AT3, AT4, AT5];

== matlab function for_elsa/Subsystem1/Subsystem1/MATLAB Function ==
  data: LRL input; MSR input; RF input; dT input; dY output; time input
function dY = fcn(LRL, MSR, RF, dT, time)

dY = ((RF/8)*(MSR-LRL)/(time*1000))*dT;
